simulink model "custom_bouncing_ball"  (R2021b)
settings: Solver=FixedStepAuto  StartTime=0.0  StopTime=10.0  RelTol=1e-3
PreLoadFcn:
  | init
undefined symbols (not defined in the file): g, r, v
settings Model: Creator=lordx  LastModifiedBy=lordx
settings HardwareCC: TargetBitPerPointer=64  TargetBitPerSizeT=64  TargetBitPerPtrDiffT=64  TargetLongLongMode=on  TargetIntDivRoundTo=Zero  TargetEndianess=LittleEndian  TargetWordSize=64  TargetHWDeviceType=MATLAB Host  ProdEqTarget=off
settings RTWCC: Description=S-Function Target with Functional Mockup Interface (FMI)  SystemTargetFile=rtwsfcnfmi.tlc  GenCodeOnly=on  GenerateMakefile=off  TemplateMakefile=rtwsfcnfmi_tmf  GenerateReport=on  LaunchReport=on  RTWCompilerOptimization=on
settings STFCustomTargetCC: TargetLangStandard=C99 (ISO)  ModelReferenceCompliant=off  CompOptLevelCompliant=on  MATLABClassNameForMDSCustomization=Simulink.SoftwareTarget.TargetSpecificTriggerConfigurationBase  SystemTargetFile=rtwsfcnfmi.tlc

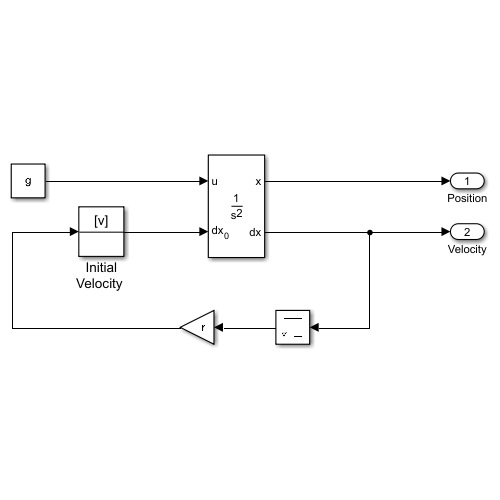
[thumbnail: Simulink's stored preview of the top-level diagram]
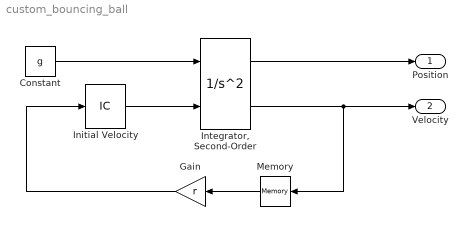
== system custom_bouncing_ball ==
  Constant : Constant  Value=g
  Gain : Gain  Gain=r
  "Initial Velocity " : InitialCondition  Value=v
  "Integrator, Second-Order" : SecondOrderIntegrator  ICSourceDXDT=external
  Memory : Memory
  Position : Outport
  Velocity : Outport  Port=2
  wires:
  "Initial Velocity "/1 -> "Integrator, Second-Order"/2
  Constant/1 -> "Integrator, Second-Order"/1
  "Integrator, Second-Order"/2 -> Memory/1, Velocity/1
  "Integrator, Second-Order"/1 -> Position/1
  Memory/1 -> Gain/1
  Gain/1 -> "Initial Velocity "/1
